simulink model "circuitoRLC"  (R2020b)
settings: Solver=VariableStepAuto  StartTime=0.0  StopTime=10.0  RelTol=1e-3
values from neighbouring files (symbols this model uses):
  C = 1    [DSF_TP0_S332_ODE45.m]    (also in DSF_TP0_S333_ODE15s.m)
  L = 1    [DSF_TP0_S332_ODE45.m]    (also in DSF_TP0_S333_ODE15s.m)
  R = 100    [DSF_TP0_S332_ODE45.m]    (also in DSF_TP0_S333_ODE15s.m)
  U = 1    [DSF_TP0_S332_ODE45.m]    (also in DSF_TP0_S333_ODE15s.m)
  y0 = [1 0]'    [DSF_TP0_S24.m]    (also in DSF_TP0_S31_FIXED.m; DSF_TP0_S32_ODE15s.m; DSF_TP0_S32_ODE45.m; DSF_TP0_S32_ODE45_DECIMADO.m)
settings Model: Creator=luis  LastModifiedBy=luis

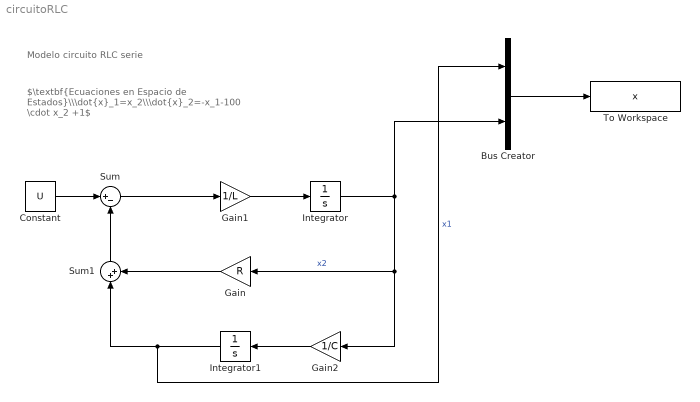
== system circuitoRLC ==
  note: Modelo circuito RLC serie
  note: $\textbf{Ecuaciones en Espacio de Estados}\\\dot{x}_1=x_2\\\dot{x}_2=-x_1-100 \cdot x_2 +1$
  Bus Creator : BusCreator  Inputs=2
  Constant : Constant  Value=U
  Gain : Gain  Gain=R
  Gain1 : Gain  Gain=1/L
  Gain2 : Gain  Gain=1/C
  Integrator : Integrator  InitialCondition=y0(2)
  Integrator1 : Integrator  InitialCondition=y0(1)
  Sum : Sum  Inputs=|+-
  Sum1 : Sum  Inputs=|++
  To Workspace : ToWorkspace  VariableName=x  SaveFormat=Timeseries  SampleTime=-1
  wires:
  Sum/1 -> Gain1/1
  Bus Creator/1 -> To Workspace/1
  Gain/1 -> Sum1/2
  Sum1/1 -> Sum/2
  Integrator/1 -> Bus Creator/2, Gain2/1, Gain/1  "x2"
  Integrator1/1 -> Bus Creator/1, Sum1/1  "x1"
  Gain1/1 -> Integrator/1
  Gain2/1 -> Integrator1/1
  Constant/1 -> Sum/1
